simulink model "ex_bus_ports_org"  (Simulink 10.0)
settings: Solver=VariableStepAuto  StartTime=0.0  StopTime=10.0  RelTol=1e-3
settings Model: Creator=The MathWorks, Inc.  LastModifiedBy=bhisma
settings DataIOCC: SaveFormat=Dataset  ReturnWorkspaceOutputs=on
settings OptimizationCC: LifeSpan=auto
settings DebuggingCC: UnderspecifiedInitializationDetection=Simplified  MergeDetectMultiDrivingBlocksExec=error  PregeneratedLibrarySubsystemCodeDiagnostic=none  SFUnexpectedBacktrackingDiag=error  SFNoUnconditionalDefaultTransitionDiag=error  SFExecutionAtInitializationDiag=warning
settings HardwareCC: ProdBitPerPointer=64  ProdBitPerSizeT=64  ProdBitPerPtrDiffT=64  ProdLargestAtomicFloat=Float  ProdIntDivRoundTo=Zero  ProdEndianess=LittleEndian  ProdWordSize=64  ProdHWDeviceType=Intel->x86-64 (Windows64)
settings ModelReferenceCC: PropagateSignalLabelsOutOfModel=on
settings GRTTargetCC: TargetLangStandard=C99 (ISO)  CombineOutputUpdateFcns=on  GRTInterface=off
settings ConfigComp: CovMetricSettings=dwe  CovHtmlReporting=off  CovSaveCumulativeToWorkspaceVar=off  CovSaveSingleToWorkspaceVar=off

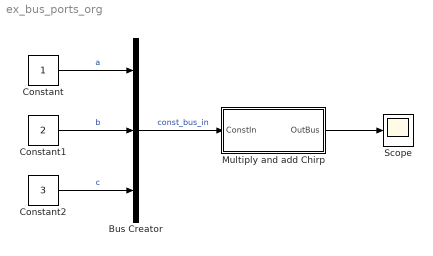
== system ex_bus_ports_org ==
  Bus Creator : BusCreator  Inputs=3
  Constant : Constant
  Constant1 : Constant  Value=2
  Constant2 : Constant  Value=3
  Multiply and add Chirp : Subsystem
  Scope : Scope
  wires:
  Constant/1 -> Bus Creator/1  "a"
  Constant1/1 -> Bus Creator/2  "b"
  Constant2/1 -> Bus Creator/3  "c"
  Bus Creator/1 -> Multiply and add Chirp/1(ConstIn)  "const_bus_in"
  Multiply and add Chirp/1(OutBus) -> Scope/1

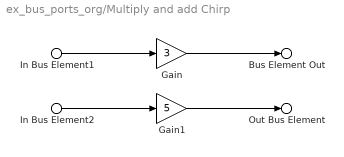
== system ex_bus_ports_org/Multiply and add Chirp ==
  In Bus Element1 : Inport  PortName=ConstIn  Element=a
  In Bus Element2 : Inport  PortName=ConstIn  Element=b
  Gain : Gain  Gain=3
  Gain1 : Gain  Gain=5
  Bus Element Out : Outport  VectorParamsAs1DForOutWhenUnconnected=off  PortName=OutBus  Element=a*3
  Out Bus Element : Outport  VectorParamsAs1DForOutWhenUnconnected=off  PortName=OutBus  Element=b*5
  wires:
  In Bus Element2/1 -> Gain1/1
  Gain/1 -> Bus Element Out/1
  Gain1/1 -> Out Bus Element/1
  In Bus Element1/1 -> Gain/1
